simulink model "van_der_pol2"  (R2015a)
settings: Solver=ode45  StartTime=0.0  StopTime=10.0  RelTol=1e-3
values from neighbouring files (symbols this model uses):
  mu = 5    [main.m]
undefined symbols (not defined in the file or in its folder): x_2
settings Model: Creator=Martin  LastModifiedBy=Martin

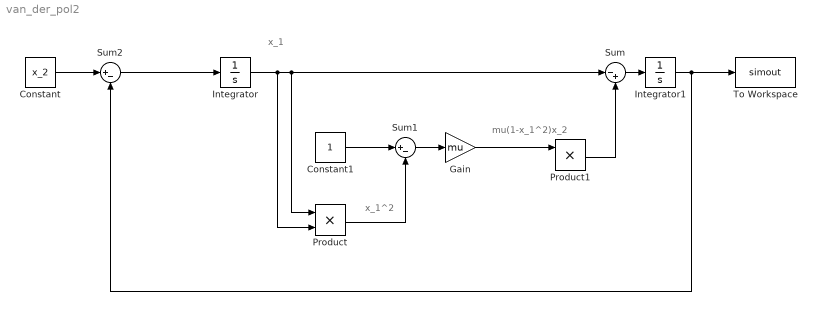
== system van_der_pol2 ==
  note: mu(1-x_1^2)x_2
  note: x_1^2
  note: x_1
  Constant : Constant  Value=x_2
  Constant1 : Constant
  Gain : Gain  Gain=mu
  Integrator : Integrator
  Integrator1 : Integrator
  Product : Product
  Product1 : Product
  Sum : Sum  Inputs=|-+
  Sum1 : Sum  Inputs=|+-
  Sum2 : Sum  Inputs=|+-
  To Workspace : ToWorkspace  VariableName=simout  SaveFormat=Timeseries  SampleTime=-1
  wires:
  Integrator/1 -> Product/2, Product/1, Sum/1
  Constant1/1 -> Sum1/1
  Product/1 -> Sum1/2
  Sum1/1 -> Gain/1
  Gain/1 -> Product1/1
  Product1/1 -> Sum/2
  Sum/1 -> Integrator1/1
  Integrator1/1 -> Sum2/2, To Workspace/1
  Constant/1 -> Sum2/1
  Sum2/1 -> Integrator/1
